simulink model "pendule_inv_capteur_etu"  (R2022a)
settings: Solver=VariableStepAuto  StartTime=0.0  StopTime=100.0  RelTol=1e-3
values from neighbouring files (symbols this model uses):
  g = 9.81    [simu_pendule_inv_capteur_etu.m]    (also in simu_pendule_inv_etu.m)
  K = [10 1]    [simu_pendule_inv_capteur_etu.m]    (also in simu_pendule_inv_etu.m)
  l = 10    [simu_pendule_inv_capteur_etu.m]    (also in simu_pendule_inv_etu.m)
  ue = 0    [simu_pendule_inv_capteur_etu.m]    (also in simu_pendule_inv_etu.m)
  x0 = [pi/20 0]'    [simu_pendule_inv_capteur_etu.m]    (also in simu_pendule_inv_etu.m)
  xe = [0 0]'    [simu_pendule_inv_capteur_etu.m]    (also in simu_pendule_inv_etu.m)
settings Model: Creator=acanon  LastModifiedBy=acanon

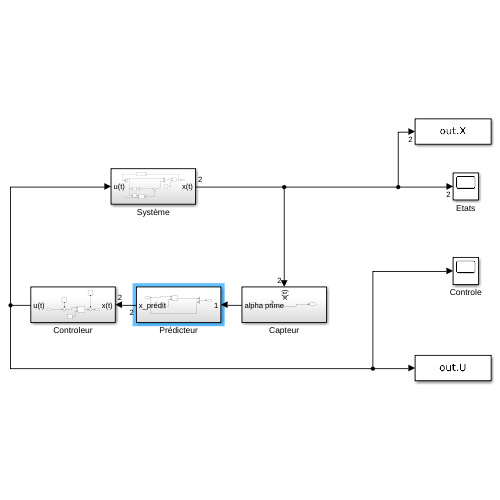
[thumbnail: Simulink's stored preview of the top-level diagram]
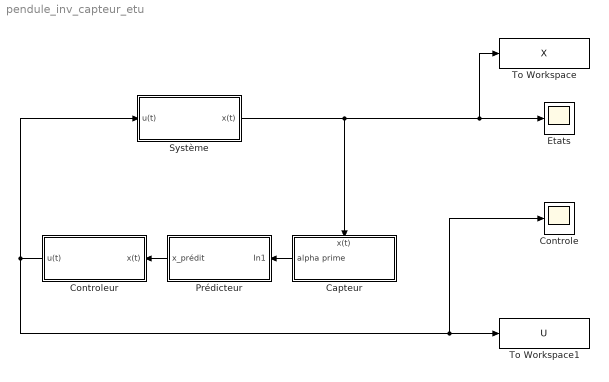
== system pendule_inv_capteur_etu ==
  Capteur : Subsystem
      settings: PortSchema="{\"entries\":[{\"content\":{\"sides\":[{\"content\":{\"connectorIds\":[]},\"type\":\"ConnectorPlacement.EquallySpacedRectSide\",\"uuid\":\"55917e7c-50a2-4d55-9b01-6b24f62dcf1b\"},{\"content\":{\"connectorIds\":[\"Out1\"],\"side\":\"RIGHT\"},\"type\":\"ConnectorPlacement.EquallySpacedRectSide\",\"uuid\":\"a02dadc6-169d-4f04-be32-da4ea2654498\"},{\"content\":{\"connectorIds\":[\"In1\"],\"side\":\"TOP\"},\"type\":\"ConnectorPlacement.EquallySpacedRectSide\",\"uuid\":\"7e0d8ce6-b3c5-446a-93c6-962789efebcf\"}]},\"type\":\"ConnectorPlacement.EquallySpacedConnector\",\"uuid\":\"32833676-defa-4a7b-854d-ac3cd35c7fe5\"}],\"packageUris\":[\"http://schema.mathworks.com/mf0/Connector/R2020b\"],\"version\":\"1.0\"}"
  Controle : Scope
  Controleur : Subsystem
  Etats : Scope
  Prédicteur : Subsystem
  Système : Subsystem
  To Workspace : ToWorkspace  VariableName=X  SaveFormat=Timeseries  SampleTime=-1
  To Workspace1 : ToWorkspace  VariableName=U  SaveFormat=Timeseries  SampleTime=-1
  wires:
  Controleur/1(u(t)) -> Système/1(u(t)), Controle/1, To Workspace1/1
  Système/1(x(t)) -> Capteur/1(x(t)), To Workspace/1, Etats/1
  Prédicteur/1(x_prédit) -> Controleur/1(x(t))
  Capteur/1(alpha prime) -> Prédicteur/1(In1)

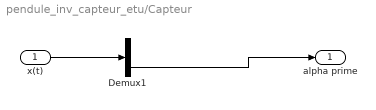
== system pendule_inv_capteur_etu/Capteur ==
  x(t) : Inport
  Demux1 : Demux  Outputs=2
  alpha prime : Outport
  wires:
  x(t)/1 -> Demux1/1
  Demux1/2 -> alpha prime/1

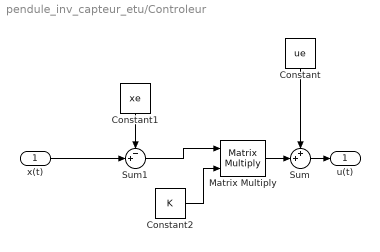
== system pendule_inv_capteur_etu/Controleur ==
  x(t) : Inport
  Constant : Constant  Value=ue
  Constant1 : Constant  Value=xe
  Constant2 : Constant  Value=K
  Matrix Multiply : Product  Multiplication=Matrix(*)
  Sum : Sum  Inputs=++|
  Sum1 : Sum  Inputs=-+|
  u(t) : Outport
  wires:
  Constant/1 -> Sum/1
  x(t)/1 -> Sum1/2
  Sum/1 -> u(t)/1
  Matrix Multiply/1 -> Sum/2
  Constant1/1 -> Sum1/1
  Constant2/1 -> Matrix Multiply/2
  Sum1/1 -> Matrix Multiply/1

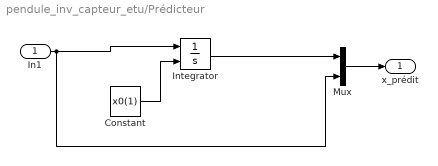
== system pendule_inv_capteur_etu/Prédicteur ==
  In1 : Inport
  Constant : Constant  Value=x0(1)
  Integrator : Integrator  InitialConditionSource=external
  Mux : Mux  Inputs=2
  x_prédit : Outport
  wires:
  In1/1 -> Mux/2, Integrator/1
  Constant/1 -> Integrator/2
  Integrator/1 -> Mux/1
  Mux/1 -> x_prédit/1

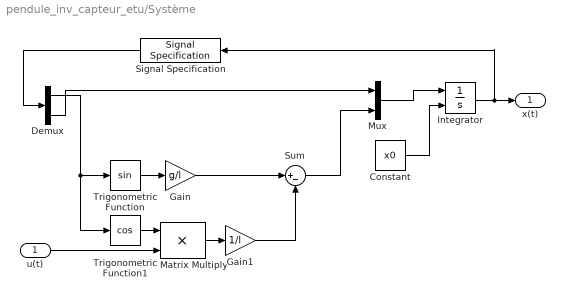
== system pendule_inv_capteur_etu/Système ==
  u(t) : Inport
  Constant : Constant  Value=x0
  Demux : Demux  Outputs=2
  Gain : Gain  Gain=g/l
  Gain1 : Gain  Gain=1/l
  Integrator : Integrator  InitialConditionSource=external
  Matrix Multiply : Product
  Mux : Mux  Inputs=2
  Signal Specification : SignalSpecification  Dimensions=2
  Sum : Sum  Inputs=|+-
  Trigonometric Function : Trigonometry
  Trigonometric Function1 : Trigonometry  Operator=cos
  x(t) : Outport
  wires:
  Demux/2 -> Mux/1
  Demux/1 -> Trigonometric Function1/1, Trigonometric Function/1
  Trigonometric Function/1 -> Gain/1
  u(t)/1 -> Matrix Multiply/2
  Trigonometric Function1/1 -> Matrix Multiply/1
  Matrix Multiply/1 -> Gain1/1
  Gain/1 -> Sum/1
  Gain1/1 -> Sum/2
  Sum/1 -> Mux/2
  Mux/1 -> Integrator/1
  Constant/1 -> Integrator/2
  Integrator/1 -> Signal Specification/1, x(t)/1
  Signal Specification/1 -> Demux/1
